simulink model "Node_M"  (R2024b)
settings: Solver=ode1  StartTime=0.0  StopTime=10.0  FixedStep=0.5e-3  RelTol=1e-3
libraries: simulink x1
settings Model: Creator=wai484  LastModifiedBy=wai484
settings SolverCC: EnableFixedStepZeroCrossing=on
settings DataIOCC: SaveOutput=off  SaveTime=off
settings ModelReferenceCC: ModelReferenceMinAlgLoopOccurrences=on
settings GRTTargetCC: CombineOutputUpdateFcns=off

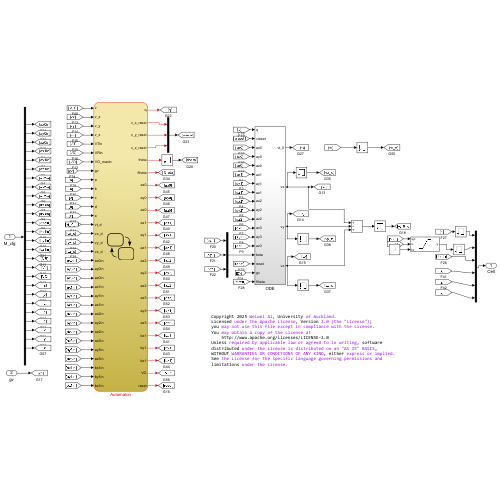
[thumbnail: Simulink's stored preview of the top-level diagram]
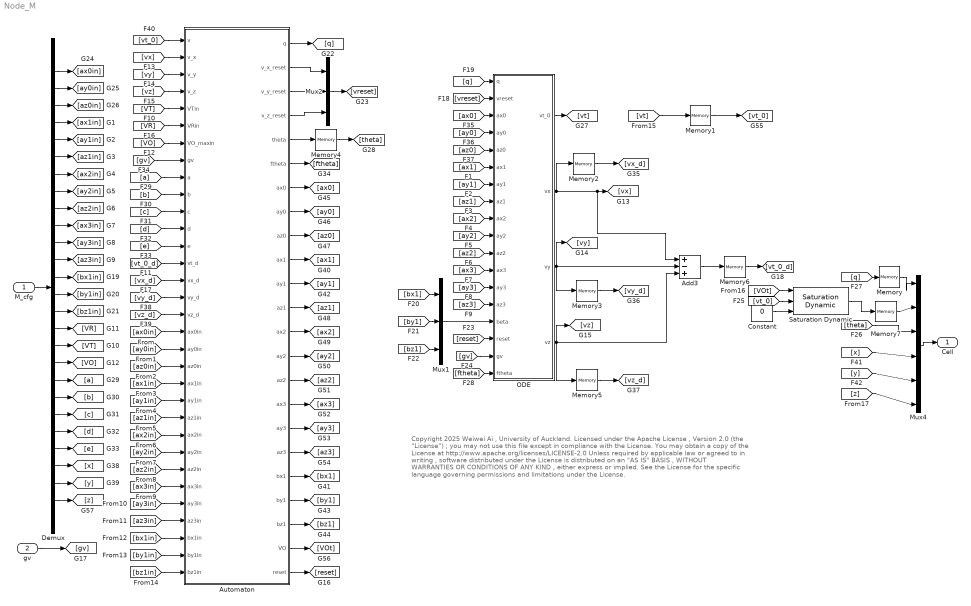
== system Node_M ==
  note: Copyright 2025 Weiwei Ai , University of Auckland.
      | Licensed under the Apache License , Version 2.0 (the "License") ;
      | you may not use this file except in compliance with the License.
      | You may obtain a copy of the License at
      | http://www.apache.org/licenses/LICENSE-2.0
      | Unless required by applicable law or agreed to in writing , software
      | distributed under the License is distributed on an "AS IS" BASIS ,
      | WITHOUT WARRANTIES OR CONDITIONS OF ANY KIND , either express or implied.
      | See the License for the specific language governing permissions and
      | limitations under the License.
  M_cfg : Inport  OutDataTypeStr=double
  gv : Inport  Port=2  OutDataTypeStr=double  PortDimensions=1
  Add3 : Sum  Inputs=+-+
  Automaton : Stateflow chart  TreatAsAtomicUnit=on
  Constant : Constant  Value=0
  Demux : Demux  Outputs=26
  Memory : Memory
  Memory{1..3,5..7} (6 alike) : Memory  InheritSampleTime=on  LinearizeAsDelay=on
  Memory4 : Memory
  Mux1 : Mux  Inputs=3
  Mux2 : Mux  Inputs=3
  Mux4 : Mux  Inputs=6
  ODE : Subsystem
  Saturation Dynamic : simulink/Discontinuities/Saturation Dynamic  OutMin=[]  OutMax=[]  OutDataTypeStr=Inherit: Same as second input  OutDataType=fixdt(1, 16)  OutScaling=2^-10  DoSatur=off
  Cell : Outport  OutDataTypeStr=double
  wires:
  M_cfg/1 -> Demux/1
  Automaton/2(v_x_reset) -> Mux2/1
  Automaton/3(v_y_reset) -> Mux2/2
  Automaton/4(v_z_reset) -> Mux2/3
  Mux4/1 -> Cell/1
  Demux/1 -> [ax0in]
  [ax0] -> ODE/3(ax0)
  Demux/2 -> [ay0in]
  [ay0] -> ODE/4(ay0)
  [az0] -> ODE/5(az0)
  Demux/3 -> [az0in]
  [ay1] -> ODE/7(ay1)
  [az1] -> ODE/8(az1)
  [ax2] -> ODE/9(ax2)
  [ay2] -> ODE/10(ay2)
  [az2] -> ODE/11(az2)
  [ax3] -> ODE/12(ax3)
  [ay3] -> ODE/13(ay3)
  [az3] -> ODE/14(az3)
  Demux/4 -> [ax1in]
  Demux/5 -> [ay1in]
  Demux/6 -> [az1in]
  Demux/7 -> [ax2in]
  Demux/8 -> [ay2in]
  Demux/9 -> [az2in]
  Demux/10 -> [ax3in]
  Demux/11 -> [ay3in]
  Demux/12 -> [az3in]
  [VT] -> Automaton/5(VTin)
  [VR] -> Automaton/6(VRin)
  Demux/18 -> [VO]
  [VO] -> Automaton/7(VO_maxin)
  ODE/2(vx) -> [vx], Add3/1, Memory2/1
  ODE/3(vy) -> [vy], Memory3/1, Add3/2
  ODE/4(vz) -> [vz], Memory5/1, Add3/3
  [vx] -> Automaton/2(v_x)
  [vy] -> Automaton/3(v_y)
  [vz] -> Automaton/4(v_z)
  [bx1] -> Mux1/1
  [by1] -> Mux1/2
  [bz1] -> Mux1/3
  Mux1/1 -> ODE/15(beta)
  Demux/13 -> [bx1in]
  Demux/14 -> [by1in]
  Demux/15 -> [bz1in]
  Demux/16 -> [VR]
  Demux/17 -> [VT]
  Automaton/23(reset) -> [reset]
  [reset] -> ODE/16(reset)
  [gv] -> ODE/17(gv)
  Mux2/1 -> [vreset]
  [vreset] -> ODE/2(vreset)
  Automaton/1(q) -> [q]
  [q] -> ODE/1(q)
  ODE/1(vt_0) -> [vt]
  Memory/1 -> Mux4/1
  [q] -> Memory/1
  [theta] -> Mux4/3
  Demux/19 -> [a]
  Demux/20 -> [b]
  Demux/21 -> [c]
  Demux/22 -> [d]
  Demux/23 -> [e]
  [ax1] -> ODE/6(ax1)
  Memory4/1 -> [theta]
  [ftheta] -> ODE/18(ftheta)
  [a] -> Automaton/9(a)
  [b] -> Automaton/10(b)
  [c] -> Automaton/11(c)
  [d] -> Automaton/12(d)
  [e] -> Automaton/13(e)
  Automaton/5(theta) -> Memory4/1
  Automaton/6(ftheta) -> [ftheta]
  Memory2/1 -> [vx_d]
  Memory3/1 -> [vy_d]
  Memory5/1 -> [vz_d]
  [vt_0_d] -> Automaton/14(vt_d)
  [vx_d] -> Automaton/15(vx_d)
  [vy_d] -> Automaton/16(vy_d)
  [vz_d] -> Automaton/17(vz_d)
  [vt_0] -> Automaton/1(v)
  Demux/24 -> [x]
  Demux/25 -> [y]
  [x] -> Mux4/4
  [y] -> Mux4/5
  [gv] -> Automaton/8(gv)
  Automaton/21(bz1) -> [bz1]
  Automaton/20(by1) -> [by1]
  Automaton/19(bx1) -> [bx1]
  Automaton/18(az3) -> [az3]
  Automaton/7(ax0) -> [ax0]
  Automaton/8(ay0) -> [ay0]
  Automaton/9(az0) -> [az0]
  Automaton/10(ax1) -> [ax1]
  Automaton/11(ay1) -> [ay1]
  Automaton/12(az1) -> [az1]
  Automaton/13(ax2) -> [ax2]
  Automaton/14(ay2) -> [ay2]
  Automaton/16(ax3) -> [ax3]
  Automaton/15(az2) -> [az2]
  [ax0in] -> Automaton/18(ax0in)
  [ay0in] -> Automaton/19(ay0in)
  [az0in] -> Automaton/20(az0in)
  [ax1in] -> Automaton/21(ax1in)
  [ay1in] -> Automaton/22(ay1in)
  [az1in] -> Automaton/23(az1in)
  [az2in] -> Automaton/26(az2in)
  [ax2in] -> Automaton/24(ax2in)
  [ay2in] -> Automaton/25(ay2in)
  Automaton/17(ay3) -> [ay3]
  [az3in] -> Automaton/29(az3in)
  [ay3in] -> Automaton/28(ay3in)
  [ax3in] -> Automaton/27(ax3in)
  [bz1in] -> Automaton/32(bz1in)
  [bx1in] -> Automaton/30(bx1in)
  [by1in] -> Automaton/31(by1in)
  Automaton/22(VO) -> [VOt]
  [vt] -> Memory1/1
  Memory1/1 -> [vt_0]
  Memory6/1 -> [vt_0_d]
  Add3/1 -> Memory6/1
  [vt_0] -> Saturation Dynamic/2
  [VOt] -> Saturation Dynamic/1
  Constant/1 -> Saturation Dynamic/3
  Memory7/1 -> Mux4/2
  Saturation Dynamic/1 -> Memory7/1
  Demux/26 -> [z]
  [z] -> Mux4/6
  gv/1 -> [gv]

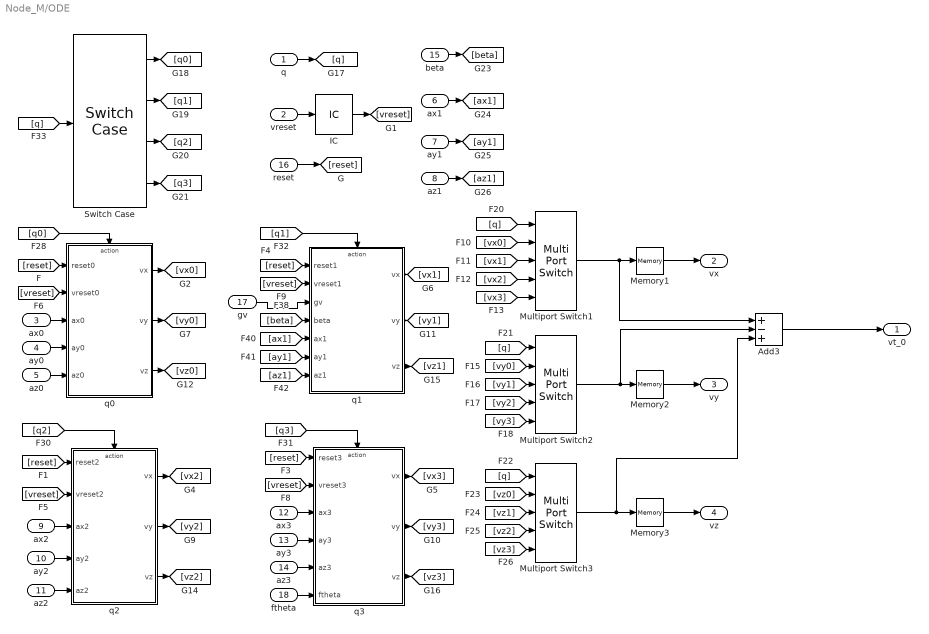
== system Node_M/ODE ==
  q : Inport
  vreset : Inport  Port=2
  ax0 : Inport  Port=3
  ay0 : Inport  Port=4
  az0 : Inport  Port=5
  ax1 : Inport  Port=6
  ay1 : Inport  Port=7
  az1 : Inport  Port=8
  ax2 : Inport  Port=9
  ay2 : Inport  Port=10
  az2 : Inport  Port=11
  ax3 : Inport  Port=12
  ay3 : Inport  Port=13
  az3 : Inport  Port=14
  beta : Inport  Port=15
  reset : Inport  Port=16
  gv : Inport  Port=17
  ftheta : Inport  Port=18
  Add3 : Sum  Inputs=+-+
  IC : InitialCondition  Value=0
  Memory1 : Memory
  Memory2 : Memory
  Memory3 : Memory
  Multiport Switch1 : MultiPortSwitch  DataPortOrder=Zero-based contiguous  Inputs=4  zeroidx=on  SaturateOnIntegerOverflow=off  InputSameDT=off
  Multiport Switch2 : MultiPortSwitch  DataPortOrder=Zero-based contiguous  Inputs=4  zeroidx=on  SaturateOnIntegerOverflow=off  InputSameDT=off
  Multiport Switch3 : MultiPortSwitch  DataPortOrder=Zero-based contiguous  Inputs=4  zeroidx=on  SaturateOnIntegerOverflow=off  InputSameDT=off
  Switch Case : SwitchCase  CaseConditions={0,1,2,3}  ShowDefaultCase=off
  q0 : Subsystem  TreatAsAtomicUnit=on
  q1 : Subsystem  TreatAsAtomicUnit=on
  q2 : Subsystem  TreatAsAtomicUnit=on
  q3 : Subsystem  TreatAsAtomicUnit=on
  vt_0 : Outport
  vx : Outport  Port=2
  vy : Outport  Port=3
  vz : Outport  Port=4
  wires:
  az3/1 -> q3/5(az3)
  [az1] -> q1/7(az1)
  [ay1] -> q1/6(ay1)
  [ax1] -> q1/5(ax1)
  [beta] -> q1/4(beta)
  beta/1 -> [beta]
  ax1/1 -> [ax1]
  ay1/1 -> [ay1]
  az1/1 -> [az1]
  [q] -> Switch Case/1
  [q1] -> q1/Action
  [q3] -> q3/Action
  [q2] -> q2/Action
  [q0] -> q0/Action
  Switch Case/4 -> [q3]
  Switch Case/3 -> [q2]
  Switch Case/2 -> [q1]
  Switch Case/1 -> [q0]
  Multiport Switch3/1 -> Memory3/1, Add3/3
  [vz3] -> Multiport Switch3/5
  [vz2] -> Multiport Switch3/4
  [vz1] -> Multiport Switch3/3
  [vz0] -> Multiport Switch3/2
  [q] -> Multiport Switch3/1
  [q] -> Multiport Switch2/1
  [q] -> Multiport Switch1/1
  [vy3] -> Multiport Switch2/5
  [vy2] -> Multiport Switch2/4
  [vy1] -> Multiport Switch2/3
  [vy0] -> Multiport Switch2/2
  [vx3] -> Multiport Switch1/5
  [vx2] -> Multiport Switch1/4
  [vx1] -> Multiport Switch1/3
  [vx0] -> Multiport Switch1/2
  q1/3(vz) -> [vz1]
  q1/2(vy) -> [vy1]
  q1/1(vx) -> [vx1]
  q3/3(vz) -> [vz3]
  q3/2(vy) -> [vy3]
  q3/1(vx) -> [vx3]
  q2/2(vy) -> [vy2]
  q2/1(vx) -> [vx2]
  q2/3(vz) -> [vz2]
  q0/3(vz) -> [vz0]
  q0/2(vy) -> [vy0]
  q0/1(vx) -> [vx0]
  [vreset] -> q1/2(vreset1)
  [vreset] -> q3/2(vreset3)
  [vreset] -> q0/2(vreset0)
  [vreset] -> q2/2(vreset2)
  [reset] -> q1/1(reset1)
  [reset] -> q3/1(reset3)
  [reset] -> q2/1(reset2)
  [reset] -> q0/1(reset0)
  ftheta/1 -> q3/6(ftheta)
  ax3/1 -> q3/3(ax3)
  Add3/1 -> vt_0/1
  ax2/1 -> q2/3(ax2)
  q/1 -> [q]
  ax0/1 -> q0/3(ax0)
  reset/1 -> [reset]
  ay0/1 -> q0/4(ay0)
  az0/1 -> q0/5(az0)
  ay2/1 -> q2/4(ay2)
  az2/1 -> q2/5(az2)
  ay3/1 -> q3/4(ay3)
  Memory1/1 -> vx/1
  Memory2/1 -> vy/1
  Memory3/1 -> vz/1
  vreset/1 -> IC/1
  IC/1 -> [vreset]
  Multiport Switch1/1 -> Memory1/1, Add3/1
  Multiport Switch2/1 -> Memory2/1, Add3/2
  gv/1 -> q1/3(gv)

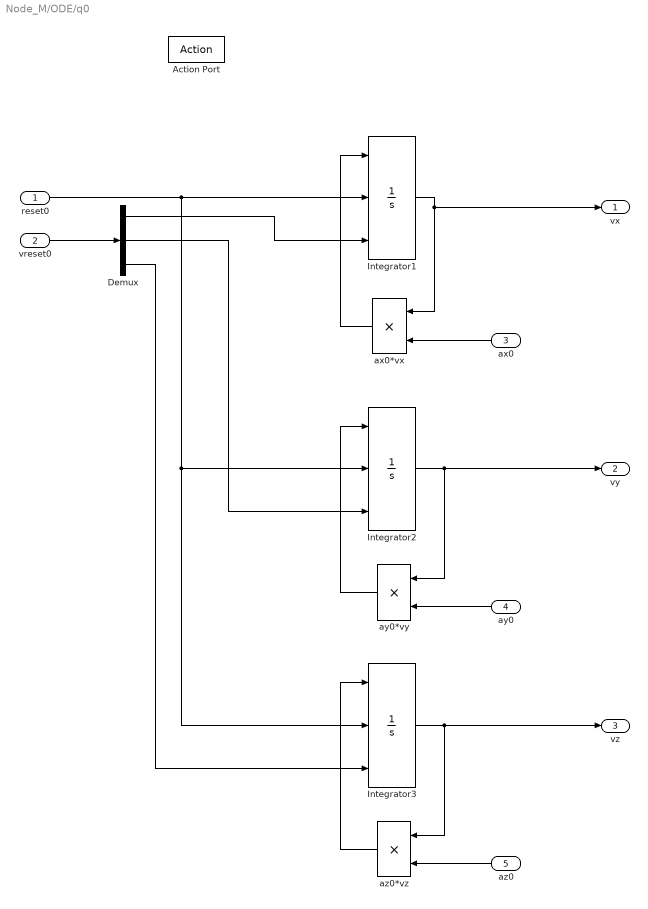
== system Node_M/ODE/q0 ==
  reset0 : Inport
  vreset0 : Inport  Port=2
  ax0 : Inport  Port=3
  ay0 : Inport  Port=4
  az0 : Inport  Port=5
  Action Port : ActionPort  InitializeStates=reset  ActionPortLabel=case [ 0 ]:
  Demux : Demux  Outputs=3
  Integrator1 : Integrator  ExternalReset=either  InitialConditionSource=external  InitialCondition=20
  Integrator2 : Integrator  ExternalReset=either  InitialConditionSource=external  InitialCondition=20
  Integrator3 : Integrator  ExternalReset=either  InitialConditionSource=external  InitialCondition=20
  ax0*vx : Product
  ay0*vy : Product
  az0*vz : Product
  vx : Outport
  vy : Outport  Port=2
  vz : Outport  Port=3
  wires:
  reset0/1 -> Integrator3/2, Integrator2/2, Integrator1/2
  ax0*vx/1 -> Integrator1/1
  Integrator1/1 -> ax0*vx/1, vx/1
  Integrator2/1 -> ay0*vy/1, vy/1
  ay0*vy/1 -> Integrator2/1
  Integrator3/1 -> vz/1, az0*vz/1
  az0*vz/1 -> Integrator3/1
  vreset0/1 -> Demux/1
  Demux/1 -> Integrator1/3
  Demux/2 -> Integrator2/3
  Demux/3 -> Integrator3/3
  ax0/1 -> ax0*vx/2
  ay0/1 -> ay0*vy/2
  az0/1 -> az0*vz/2

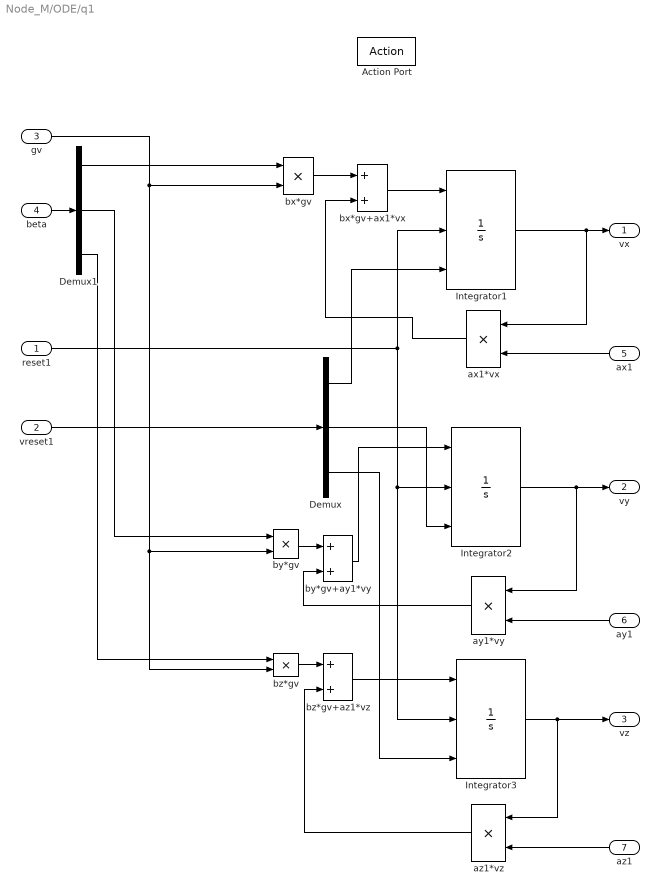
== system Node_M/ODE/q1 ==
  reset1 : Inport
  vreset1 : Inport  Port=2
  gv : Inport  Port=3
  beta : Inport  Port=4
  ax1 : Inport  Port=5
  ay1 : Inport  Port=6
  az1 : Inport  Port=7
  Action Port : ActionPort  InitializeStates=reset  ActionPortLabel=case [ 1 ]:
  Demux : Demux  Outputs=3
  Demux1 : Demux  Outputs=3
  Integrator1 : Integrator  ExternalReset=either  InitialConditionSource=external  InitialCondition=1
  Integrator2 : Integrator  ExternalReset=either  InitialConditionSource=external  InitialCondition=1
  Integrator3 : Integrator  ExternalReset=either  InitialConditionSource=external  InitialCondition=1
  ax1*vx : Product
  ay1*vy : Product
  az1*vz : Product
  bx*gv : Product
  bx*gv+ax1*vx : Sum
  by*gv : Product
  by*gv+ay1*vy : Sum
  bz*gv : Product
  bz*gv+az1*vz : Sum
  vx : Outport
  vy : Outport  Port=2
  vz : Outport  Port=3
  wires:
  Demux1/3 -> bz*gv/1
  Demux1/1 -> bx*gv/1
  beta/1 -> Demux1/1
  vreset1/1 -> Demux/1
  Integrator3/1 -> az1*vz/1, vz/1
  Integrator2/1 -> ay1*vy/1, vy/1
  Integrator1/1 -> vx/1, ax1*vx/1
  gv/1 -> bx*gv/2, by*gv/2, bz*gv/2
  reset1/1 -> Integrator1/2, Integrator2/2, Integrator3/2
  Demux/1 -> Integrator1/3
  Demux/2 -> Integrator2/3
  Demux/3 -> Integrator3/3
  az1/1 -> az1*vz/2
  bz*gv/1 -> bz*gv+az1*vz/1
  az1*vz/1 -> bz*gv+az1*vz/2
  bz*gv+az1*vz/1 -> Integrator3/1
  ay1/1 -> ay1*vy/2
  ay1*vy/1 -> by*gv+ay1*vy/2
  by*gv/1 -> by*gv+ay1*vy/1
  by*gv+ay1*vy/1 -> Integrator2/1
  bx*gv+ax1*vx/1 -> Integrator1/1
  ax1/1 -> ax1*vx/2
  bx*gv/1 -> bx*gv+ax1*vx/1
  ax1*vx/1 -> bx*gv+ax1*vx/2
  Demux1/2 -> by*gv/1

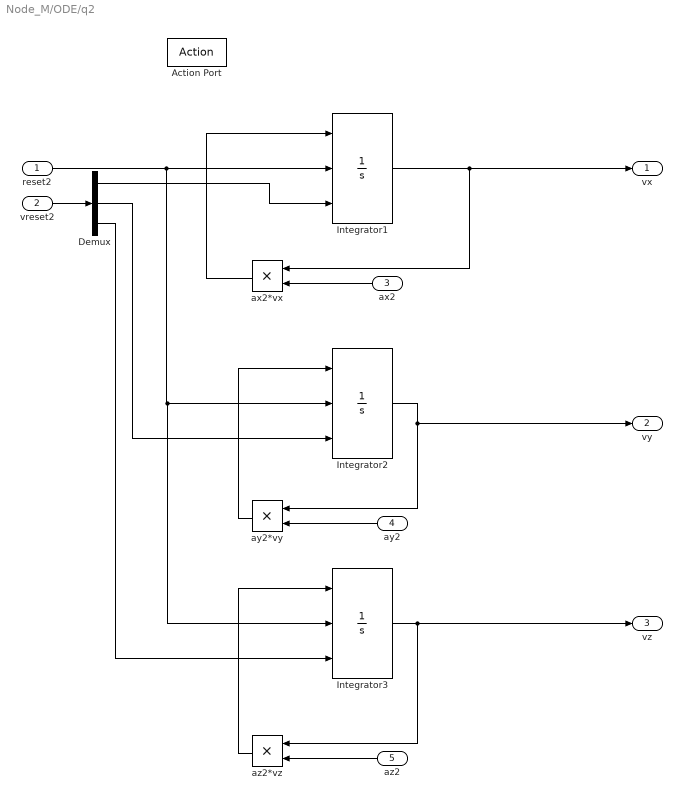
== system Node_M/ODE/q2 ==
  reset2 : Inport
  vreset2 : Inport  Port=2
  ax2 : Inport  Port=3
  ay2 : Inport  Port=4
  az2 : Inport  Port=5
  Action Port : ActionPort  InitializeStates=reset  ActionPortLabel=case [ 2 ]:
  Demux : Demux  Outputs=3
  Integrator1 : Integrator  ExternalReset=either  InitialConditionSource=external  InitialCondition=20
  Integrator2 : Integrator  ExternalReset=either  InitialConditionSource=external  InitialCondition=20
  Integrator3 : Integrator  ExternalReset=either  InitialConditionSource=external  InitialCondition=20
  ax2*vx : Product
  ay2*vy : Product
  az2*vz : Product
  vx : Outport
  vy : Outport  Port=2
  vz : Outport  Port=3
  wires:
  reset2/1 -> Integrator3/2, Integrator2/2, Integrator1/2
  ax2*vx/1 -> Integrator1/1
  ax2/1 -> ax2*vx/2
  Integrator1/1 -> ax2*vx/1, vx/1
  Integrator2/1 -> ay2*vy/1, vy/1
  ay2/1 -> ay2*vy/2
  Integrator3/1 -> az2*vz/1, vz/1
  az2/1 -> az2*vz/2
  ay2*vy/1 -> Integrator2/1
  az2*vz/1 -> Integrator3/1
  vreset2/1 -> Demux/1
  Demux/1 -> Integrator1/3
  Demux/2 -> Integrator2/3
  Demux/3 -> Integrator3/3

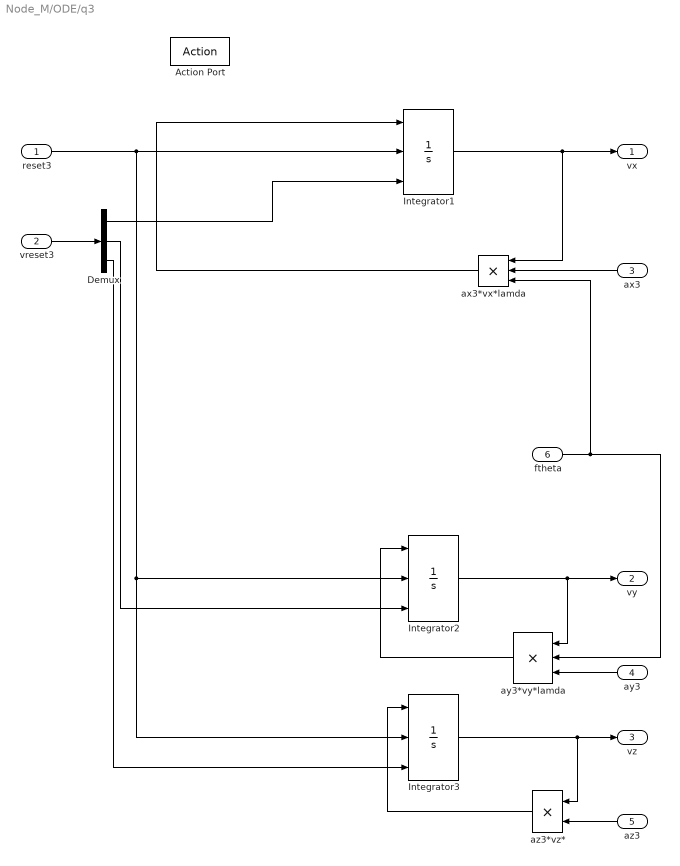
== system Node_M/ODE/q3 ==
  reset3 : Inport
  vreset3 : Inport  Port=2
  ax3 : Inport  Port=3
  ay3 : Inport  Port=4
  az3 : Inport  Port=5
  ftheta : Inport  Port=6
  Action Port : ActionPort  InitializeStates=reset  ActionPortLabel=case [ 3 ]:
  Demux : Demux  Outputs=3
  Integrator1 : Integrator  ExternalReset=either  InitialConditionSource=external  InitialCondition=133
  Integrator2 : Integrator  ExternalReset=either  InitialConditionSource=external  InitialCondition=133
  Integrator3 : Integrator  ExternalReset=either  InitialConditionSource=external  InitialCondition=133
  ax3*vx*lamda : Product  Inputs=3
  ay3*vy*lamda : Product  Inputs=3
  az3*vz* : Product
  vx : Outport
  vy : Outport  Port=2
  vz : Outport  Port=3
  wires:
  ftheta/1 -> ax3*vx*lamda/3, ay3*vy*lamda/2
  reset3/1 -> Integrator3/2, Integrator2/2, Integrator1/2
  ax3*vx*lamda/1 -> Integrator1/1
  ax3/1 -> ax3*vx*lamda/2
  Integrator1/1 -> ax3*vx*lamda/1, vx/1
  ay3*vy*lamda/1 -> Integrator2/1
  Integrator2/1 -> ay3*vy*lamda/1, vy/1
  Integrator3/1 -> az3*vz*/1, vz/1
  ay3/1 -> ay3*vy*lamda/3
  az3/1 -> az3*vz*/2
  az3*vz*/1 -> Integrator3/1
  vreset3/1 -> Demux/1
  Demux/1 -> Integrator1/3
  Demux/2 -> Integrator2/3
  Demux/3 -> Integrator3/3

== stateflow chart Node_M/Automaton ==
  state Resting_FR
    en: q=0;
    VT=VTin;
  state Stimulated
    en: q=1;
  state Plateau_ER
    en:q=3;
  state Upstroke
    en: q=2;
  (default) -> Resting_FR : {[ax0,ay0,az0,ax1,ay1,az1,ax2,ay2,az2,ax3,ay3,az3,bx1,by1,bz1]=pupdate;}
  Resting_FR -> Stimulated : [(gv>VT)&&v<=VT]{...
      | [ax0,ay0,az0,ax1,ay1,az1,ax2,ay2,az2,ax3,ay3,az3,bx1,by1,bz1]=pupdate;
      | VO_max=VO_maxin;
      | VR=VRin;
      | v_x_reset=v_x;
      | v_y_reset=v_y;
      | v_z_reset=v_z;
      | vno=v;VO=VO_max-80.1*sqrt(vno/VR);
      | [theta,ftheta]=vtheta(vno,VR,a,b,c,d,e);
      | reset;}
  Stimulated -> Resting_FR [order 2] : [(gv<=0)&&v<VT]{...
      | v_x_reset=v_x;
      | v_y_reset=v_y;
      | v_z_reset=v_z;
      | reset;}
  Stimulated -> Upstroke [order 1] : [v>=VT]{...
      | v_x_reset=(v_x-vx_d)*(VT-vt_d)/(v-vt_d)+vx_d;
      | v_y_reset=(v_y-vy_d)*(VT-vt_d)/(v-vt_d)+vy_d;
      | v_z_reset=(v_z-vz_d)*(VT-vt_d)/(v-vt_d)+vz_d;
      | reset;}
  Plateau_ER -> Resting_FR : [v<=VR]{...
      | v_x_reset=(v_x-vx_d)*(VR-vt_d)/(v-vt_d)+vx_d;
      | v_y_reset=(v_y-vy_d)*(VR-vt_d)/(v-vt_d)+vy_d;
      | v_z_reset=(v_z-vz_d)*(VR-vt_d)/(v-vt_d)+vz_d;
      | reset;}
  Upstroke -> Plateau_ER : [v>=VO]{...
      | v_x_reset=(v_x-vx_d)*(VO-vt_d)/(v-vt_d)+vx_d;
      | v_y_reset=(v_y-vy_d)*(VO-vt_d)/(v-vt_d)+vy_d;
      | v_z_reset=(v_z-vz_d)*(VO-vt_d)/(v-vt_d)+vz_d;
      | reset;}
  data: pax0 function_output double; pay0 function_output double; paz0 function_output double; pax1 function_output double; pay1 function_output double; paz1 function_output double; pax2 function_output double; pay2 function_output double; paz2 function_output double; pax3 function_output double; pay3 function_output double; paz3 function_output double; pbx1 function_output double; pby1 function_output double; pbz1 function_output double; vnin function_input double; VRi function_input double; ain function_input double; bin function_input double; cin function_input double; din function_input double; ein function_input double; thetaout function_output double; fthetatout function_output double; v input double; q output double; v_x input; v_y input; v_z input; v_x_reset output double =0; v_y_reset output double =0; v_z_reset output double =0; vno local double; VTin input; VRin input; VO_maxin input double; gv input; theta output double; ftheta output double; a input double; b input double; c input double; d input double; e input double; vt_d input double; vx_d input double; vy_d input double; vz_d input double; ax0 output; ay0 output; az0 output; ax1 output; ay1 output; az1 output; ax2 output; ay2 output; az2 output; ax3 output; ay3 output; az3 output; bx1 output; by1 output; bz1 output; ax0in input; ay0in input; az0in input; ax1in input; ay1in input; az1in input; ax2in input; ay2in input; az2in input; ax3in input; ay3in input; az3in input; bx1in input; by1in input; bz1in input; VO_max local; VR local; VT local; VO output double
  events: reset output EITHER_EDGE_EVENT
  function [pax0,pay0,paz0,pax1,pay1,paz1,pax2,pay2,paz2,pax3,pay3,paz3,pbx1,pby1,pbz1]=pupdate:
    | function [pax0,pay0,paz0,pax1,pay1,paz1,pax2,pay2,paz2,pax3,pay3,paz3,pbx1,pby1,pbz1]=pupdate
    | pax0=ax0in;
    | pay0=ay0in;
    | paz0=az0in;
    | pax1=ax1in;
    | pay1=ay1in;
    | paz1=az1in;
    | pax2=ax2in;
    | pay2=ay2in;
    | paz2=az2in;
    | pax3=ax3in;
    | pay3=ay3in;
    | paz3=az3in;
    | pbx1=bx1in;
    | pby1=by1in;
    | pbz1=bz1in;
  function [thetaout,fthetatout]  = vtheta(vnin,VRi,ain,bin,cin,din,ein):
    | function [thetaout,fthetatout]  = vtheta(vnin,VRi,ain,bin,cin,din,ein)
    | %Rate dependent factor
    | thetaout=vnin/VRi;
    | if thetaout<ein
    |     fthetatout=ain*exp(bin*thetaout)+cin*exp(-din*thetaout);
    | else
    |     fthetatout=ain*exp(bin*ein)+cin*exp(-din*ein);
    |     thetaout=ein;
    | end
    | 
    | end
